simulink model "qizhongji"  (Simulink 8.7)
settings: Solver=VariableStepAuto  StartTime=0.0  StopTime=200  RelTol=1e-3
settings Model: Creator=Administrator  LastModifiedBy=Administrator
settings DataIOCC: LimitDataPoints=off  SaveFormat=Dataset
settings DebuggingCC: UnderspecifiedInitializationDetection=Simplified  MergeDetectMultiDrivingBlocksExec=error
settings HardwareCC: ProdBitPerPointer=64  ProdLargestAtomicFloat=Float  ProdIntDivRoundTo=Zero  ProdEndianess=LittleEndian  ProdWordSize=64  ProdHWDeviceType=Intel->x86-64 (Windows64)
settings ModelReferenceCC: PropagateSignalLabelsOutOfModel=on
settings ConfigComp: CovModelRefEnable=off

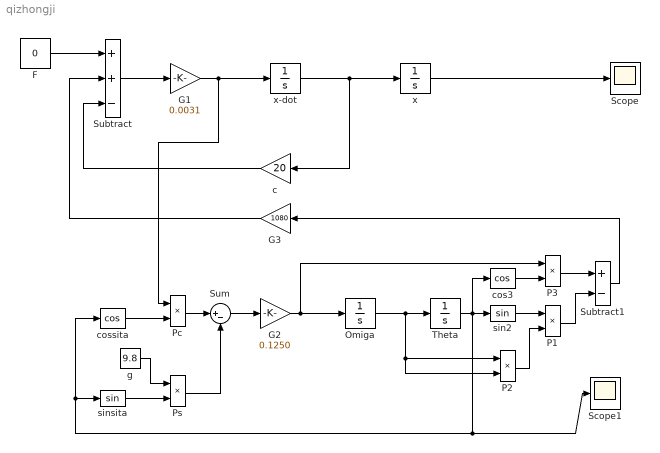
== system qizhongji ==
  F : Constant  Value=0
  G1 : Gain  Gain=0.0031
  G2 : Gain  Gain=0.1250
  G3 : Gain  Gain=1080
  Omiga : Integrator  InitialCondition=0.01
  P1 : Product
  P2 : Product
  P3 : Product
  Pc : Product
  Ps : Product
  Scope : Scope
  Scope1 : Scope
  Subtract : Sum  Inputs=++-
  Subtract1 : Sum  Inputs=+-
  Sum : Sum  Inputs=|+-
  Theta : Integrator
  c : Gain  Gain=20
  cos3 : Trigonometry  Operator=cos
  cossita : Trigonometry  Operator=cos
  g : Constant  Value=9.8
  sin2 : Trigonometry
  sinsita : Trigonometry
  x : Integrator
  x-dot : Integrator
  wires:
  F/1 -> Subtract/1
  Subtract/1 -> G1/1
  G1/1 -> x-dot/1, Pc/1
  x-dot/1 -> c/1, x/1
  x/1 -> Scope/1
  c/1 -> Subtract/3
  G3/1 -> Subtract/2
  Subtract1/1 -> G3/1
  P3/1 -> Subtract1/1
  P1/1 -> Subtract1/2
  cos3/1 -> P3/2
  sin2/1 -> P1/1
  Omiga/1 -> P2/2, P2/1, Theta/1
  G2/1 -> P3/1, Omiga/1
  P2/1 -> P1/2
  Pc/1 -> Sum/1
  Sum/1 -> G2/1
  sinsita/1 -> Ps/2
  Ps/1 -> Sum/2
  g/1 -> Ps/1
  cossita/1 -> Pc/2
  Theta/1 -> sinsita/1, cossita/1, Scope1/1, cos3/1, sin2/1
